simulink model "GridN3"  (R2021a)
settings: Solver=VariableStepAuto  StartTime=0.0  StopTime=10.0  RelTol=1e-3
libraries: spsDistributedParametersLineLib x22, spsThreePhaseSeriesRLCLoadLib x6, spsThreePhaseVIMeasurementLib x2, spspowerguiLib x1
settings Model: Creator=miair  LastModifiedBy=Admin
settings SolverCC: AlgebraicLoopSolver=TrustRegion
settings DataIOCC: ReturnWorkspaceOutputs=off
settings DebuggingCC: SFMachineParentedDataDiag=warning  ArithmeticOperatorsInVariantConditions=warning
settings SFSimCC: SimUseLocalCustomCode=off  CustomCodeUndefinedFunction=UseInterfaceOnly
settings RTWCC: RTWUseLocalCustomCode=off
settings CodeAppCC: StateflowObjectComments=on
settings SimscapeCC: SimscapeNormalizeSystem=off

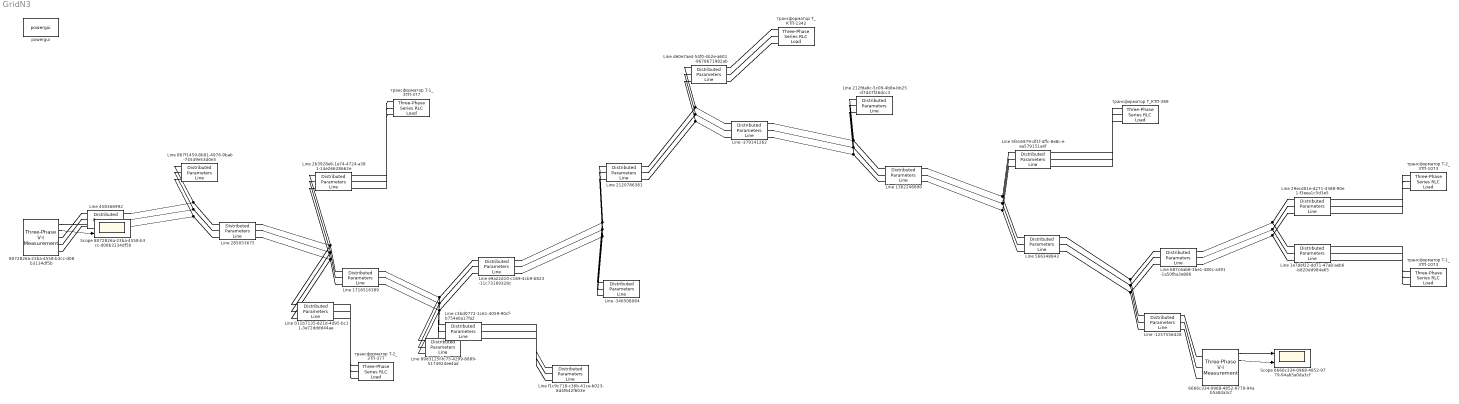
== system GridN3 ==
  6666c334-0968-4852-9779-94ab5a0da3cf : spsThreePhaseVIMeasurementLib/Three-Phase V-I Measurement  VoltageMeasurement=phase-to-ground  SetLabelV=off  LabelV=Vabc  Vpu=off  VpuLL=off  CurrentMeasurement=yes  SetLabelI=off  LabelI=Iabc  Ipu=off  Pbase=100e6  Vbase=500e3  OutputType=Complex  PhasorSimulation=on  PSBequivalent=0
  8072826a-23ba-4558-b3cc-d08b3134df5b : spsThreePhaseVIMeasurementLib/Three-Phase V-I Measurement  VoltageMeasurement=phase-to-ground  SetLabelV=off  LabelV=Vabc  Vpu=off  VpuLL=off  CurrentMeasurement=yes  SetLabelI=off  LabelI=Iabc  Ipu=off  Pbase=100e6  Vbase=500e3  OutputType=Complex  PhasorSimulation=on  PSBequivalent=0
  Line -1257556428 : spsDistributedParametersLineLib/Distributed Parameters Line  Description=Line connected to devices: [Опора-7/3_РВА-18-10кВ, ВВ РВА-19-10кВ]  Phases=3  Length=0.083645  Frequency=50  Resistance=[0.646656091154803 0.0486237908083191 0.0486712220507153;0.0486237908083191 0.646561225344642 0.0486237934466192;0.0486712220507153 0.0486237934466192 0.646656091154803]  Inductance=[0.00282448912315926 0.00133270803418135 0.00132951476746136;0.00133270803418135 0.00282479813276775 0.00133799988507366;0.00132951476746136 0.00133799988507366 0.00282448912315926]  Capacitance=[7.89543174552926e-09 -1.85986777702161e-09 -1.7901190036642e-09;-1.85986777702161e-09 7.82540023894543e-09 -1.8957321828871e-09;-1.7901190036642e-09 -1.8957321828871e-09 7.91264394645417e-09]  x1=[85.8130478893877 6561.48353456322 6560.92029844219;314.159265358979 314.159265358979 314.159265358979;0.298986720881434 -0.899555226132864 -2.47049778639167]  x2=[85.8130485695924 6561.4835673883 6560.92033132697;314.159265358979 314.159265358979 314.159265358979;0.298986717463087 -0.899555232497847 -2.47049779281051]  x3=[0.07502629314561 16.6966616361443 16.8234452112218;314.159265358979 314.159265358979 314.159265358979;0.298860809828188 -0.899655256227905 -2.47059791172944]  x4=[0.0750262931601746 16.6966616361894 16.8234452113946;314.159265358979 314.159265358979 314.159265358979;0.298986717302174 -0.899555232500781 -2.47049779281513]  x5=4.00782735046359e-07  V1=ones(3,3)  V2=ones(3,3)  I1=ones(3,3)  I2=ones(3,3)  nHarmo=1  Measurements=None  Decoupling=off  VsMag0=0  VrMag0=0  VsAngle0=0  VrAngle0=0  IsMag0=0  IrMag0=0  IsAngle0=0  IrAngle0=0
      settings: SourceProductBaseCode=PS
  Line -346508084 : spsDistributedParametersLineLib/Distributed Parameters Line  Description=Line connected to devices: [Опора-2/18_РВА-18-10кВ, трансформатор Т_ТП-1060]  Phases=3  Length=0.088705  Frequency=50  Resistance=[0.991907494602668 0.595664141602668 0.595664141602668;0.595664141602668 0.991907494602668 0.595664141602668;0.595664141602668 0.595664141602668 0.991907494602668]  Inductance=[0.0013307605340619 0.0010400448682494 0.0010400448682494;0.0010400448682494 0.0013307605340619 0.0010400448682494;0.0010400448682494 0.0010400448682494 0.0013307605340619]  Capacitance=[4.05772665830295e-07 -7.83285059789075e-08 -7.83285016498931e-08;-7.83285059789075e-08 4.05772632089447e-07 -7.83285164513028e-08;-7.83285016498931e-08 -7.83285164513028e-08 4.05772808751434e-07]  x1=[0.325825360935298 6568.42511930154 6568.48441213397;314.159265358979 314.159265358979 314.159265358979;0.746760518849295 2.95396210897823 1.38316414063238]  x2=[0.325825468435743 6568.42547824959 6568.48477108536;314.159265358979 314.159265358979 314.159265358979;0.746759846634459 2.95396187188771 1.3831639035418]  x3=[0.00278109088771278 267.749063807252 267.751511330739;314.159265358979 314.159265358979 314.159265358979;0.745947870811163 2.95363139241199 1.38283342402768]  x4=[0.00278109087609533 267.749063812641 267.751511335979;314.159265358979 314.159265358979 314.159265358979;0.746759838440762 2.95396187188745 1.38316390354211]  x5=2.58571089417873e-06  V1=ones(3,3)  V2=ones(3,3)  I1=ones(3,3)  I2=ones(3,3)  nHarmo=1  Measurements=None  Decoupling=off  VsMag0=0  VrMag0=0  VsAngle0=0  VrAngle0=0  IsMag0=0  IrMag0=0  IsAngle0=0  IrAngle0=0
      settings: SourceProductBaseCode=PS
  Line -379141262 : spsDistributedParametersLineLib/Distributed Parameters Line  Description=Line connected to devices: [Опора-2/22_РВА-18-10кВ, СШ ЗТП-921]  Phases=3  Length=0.22086  Frequency=50  Resistance=[0.646656091154803 0.0486237908083191 0.0486712220507153;0.0486237908083191 0.646561225344642 0.0486237934466192;0.0486712220507153 0.0486237934466192 0.646656091154803]  Inductance=[0.00282448912315926 0.00133270803418135 0.00132951476746136;0.00133270803418135 0.00282479813276775 0.00133799988507366;0.00132951476746136 0.00133799988507366 0.00282448912315926]  Capacitance=[7.89543174552926e-09 -1.85986777702161e-09 -1.7901190036642e-09;-1.85986777702161e-09 7.82540023894543e-09 -1.8957321828871e-09;-1.7901190036642e-09 -1.8957321828871e-09 7.91264394645417e-09]  x1=[85.7807223973082 6566.46218095662 6565.89154860446;314.159265358979 314.159265358979 314.159265358979;0.2985403295409 -0.899438697475493 -2.47038427952299]  x2=[85.7923784155305 6564.66837221298 6564.10040565809;314.159265358979 314.159265358979 314.159265358979;0.29862678418753 -0.899539931779373 -2.47048448218466]  x3=[0.104287106341695 6.82361878036728 6.92958778579486;314.159265358979 314.159265358979 314.159265358979;0.117621774807592 -0.363172627151027 -1.9436572281585]  x4=[0.0509827963357022 27.7636713522879 27.8913212019681;314.159265358979 314.159265358979 314.159265358979;0.675072542911708 -1.02556648080429 -2.59583033227613]  x5=1.0582446633073e-06  V1=ones(3,3)  V2=ones(3,3)  I1=ones(3,3)  I2=ones(3,3)  nHarmo=1  Measurements=None  Decoupling=off  VsMag0=0  VrMag0=0  VsAngle0=0  VrAngle0=0  IsMag0=0  IrMag0=0  IsAngle0=0  IrAngle0=0
      settings: SourceProductBaseCode=PS
  Line 011b7135-821d-4d95-bc11-3e72dddd44ae : spsDistributedParametersLineLib/Distributed Parameters Line  Description=Line connected to devices: [СШ ЗТП-377, трансформатор Т-2_ЗТП-377]  Phases=3  Length=0.005  Frequency=50  Resistance=[0.476003738225748 0.351747138225748 0.351747138225748;0.351747138225748 0.476003738225748 0.351747138225748;0.351747138225748 0.351747138225748 0.476003738225748]  Inductance=[0.000705954362986426 0.000459934243504405 0.000459934243504405;0.000459934243504405 0.000705954362986426 0.000459934243504405;0.000459934243504405 0.000459934243504405 0.000705954362986426]  Capacitance=[5.7561313269996e-07 -1.37543883484145e-07 -1.37543912800485e-07;-1.37543883484145e-07 5.75613027339387e-07 -1.37543875208088e-07;-1.37543912800485e-07 -1.37543875208088e-07 5.75613005057695e-07]  x1=[0.18202648425754 6574.92237471971 6574.93859363999;314.159265358979 314.159265358979 314.159265358979;0.731824412238409 -0.817080733458179 -2.38787252861853]  x2=[0.182026484492195 6574.92000203471 6574.93622094912;314.159265358979 314.159265358979 314.159265358979;0.731824413700631 -0.817080821744966 -2.38787261690532]  x3=[0.00247469117336317 350.815663562059 350.816501570652;314.159265358979 314.159265358979 314.159265358979;0.731816309663396 -0.81412926345355 -2.38492105836423]  x4=[0.0024745921934232 357.160743494514 357.161597181016;314.159265358979 314.159265358979 314.159265358979;0.731797613463593 -0.820000478759535 -2.39079227415924]  x5=1.10521588109605e-07  V1=ones(3,3)  V2=ones(3,3)  I1=ones(3,3)  I2=ones(3,3)  nHarmo=1  Measurements=None  Decoupling=off  VsMag0=0  VrMag0=0  VsAngle0=0  VrAngle0=0  IsMag0=0  IrMag0=0  IsAngle0=0  IrAngle0=0
      settings: SourceProductBaseCode=PS
  Line 1362246896 : spsDistributedParametersLineLib/Distributed Parameters Line  Description=Line connected to devices: [СШ ЗТП-921, СШ КТП-389]  Phases=3  Length=0.37012  Frequency=50  Resistance=[0.646656091154803 0.0486237908083191 0.0486712220507153;0.0486237908083191 0.646561225344642 0.0486237934466192;0.0486712220507153 0.0486237934466192 0.646656091154803]  Inductance=[0.00282448912315926 0.00133270803418135 0.00132951476746136;0.00133270803418135 0.00282479813276775 0.00133799988507366;0.00132951476746136 0.00133799988507366 0.00282448912315926]  Capacitance=[7.89543174552926e-09 -1.85986777702161e-09 -1.7901190036642e-09;-1.85986777702161e-09 7.82540023894543e-09 -1.8957321828871e-09;-1.7901190036642e-09 -1.8957321828871e-09 7.91264394645417e-09]  x1=[85.7923784155308 6564.66837221298 6564.10040565809;314.159265358979 314.159265358979 314.159265358979;0.298402105266729 -0.899718424425486 -2.47066314474314]  x2=[85.8119032777789 6561.66012948809 6561.09663330914;314.159265358979 314.159265358979 314.159265358979;0.298546930444211 -0.899887751165177 -2.47083073957211]  x3=[0.104282336760185 6.82326507299442 6.92908966322945;314.159265358979 314.159265358979 314.159265358979;0.11750414593762 -0.361669324534678 -1.94217067702694]  x4=[0.0509963380008713 27.7541994828913 27.8817464459583;314.159265358979 314.159265358979 314.159265358979;0.674503619209762 -1.02641198177557 -2.59667506905694]  x5=1.77341988039164e-06  V1=ones(3,3)  V2=ones(3,3)  I1=ones(3,3)  I2=ones(3,3)  nHarmo=1  Measurements=None  Decoupling=off  VsMag0=0  VrMag0=0  VsAngle0=0  VrAngle0=0  IsMag0=0  IrMag0=0  IsAngle0=0  IrAngle0=0
      settings: SourceProductBaseCode=PS
  Line 1716516389 : spsDistributedParametersLineLib/Distributed Parameters Line  Description=Line connected to devices: [СШ ЗТП-377, Опора-2/17_РВА-18-10кВ]  Phases=3  Length=0.75608  Frequency=50  Resistance=[0.646656091154803 0.0486237908083191 0.0486712220507153;0.0486237908083191 0.646561225344642 0.0486237934466192;0.0486712220507153 0.0486237934466192 0.646656091154803]  Inductance=[0.00282448912315926 0.00133270803418135 0.00132951476746136;0.00133270803418135 0.00282479813276775 0.00133799988507366;0.00132951476746136 0.00133799988507366 0.00282448912315926]  Capacitance=[7.89543174552926e-09 -1.85986777702161e-09 -1.7901190036642e-09;-1.85986777702161e-09 7.82540023894543e-09 -1.8957321828871e-09;-1.7901190036642e-09 -1.8957321828871e-09 7.91264394645417e-09]  x1=[85.7303472897462 6574.23848711095 6573.65682525224;314.159265358979 314.159265358979 314.159265358979;0.297343931698933 -0.899609585013276 -2.47056030786269]  x2=[85.7698176529276 6568.14269532905 6567.56961227306;314.159265358979 314.159265358979 314.159265358979;0.297652273334468 -0.899981244223213 -2.47092840739886]  x3=[0.10467535670815 6.59358891496528 6.70130181002506;314.159265358979 314.159265358979 314.159265358979;0.122437480289168 -0.392072680443273 -1.97247119055127]  x4=[0.0502114079757094 27.8421642336423 27.9697944201387;314.159265358979 314.159265358979 314.159265358979;0.667253673963557 -1.01573694491228 -2.58604709943669]  x5=3.62273668855104e-06  V1=ones(3,3)  V2=ones(3,3)  I1=ones(3,3)  I2=ones(3,3)  nHarmo=1  Measurements=None  Decoupling=off  VsMag0=0  VrMag0=0  VsAngle0=0  VrAngle0=0  IsMag0=0  IrMag0=0  IsAngle0=0  IrAngle0=0
      settings: SourceProductBaseCode=PS
  Line 1e7def22-dd71-47a8-aeb6-b820dd984e65 : spsDistributedParametersLineLib/Distributed Parameters Line  Description=Line connected to devices: [СШ ЗТП-1073, трансформатор Т-1_ЗТП-1073]  Phases=3  Length=0.005  Frequency=50  Resistance=[0.476003738225748 0.351747138225748 0.351747138225748;0.351747138225748 0.476003738225748 0.351747138225748;0.351747138225748 0.351747138225748 0.476003738225748]  Inductance=[0.000705954362986426 0.000459934243504405 0.000459934243504405;0.000459934243504405 0.000705954362986426 0.000459934243504405;0.000459934243504405 0.000459934243504405 0.000705954362986426]  Capacitance=[5.7561313269996e-07 -1.37543883484145e-07 -1.37543912800485e-07;-1.37543883484145e-07 5.75613027339387e-07 -1.37543875208088e-07;-1.37543912800485e-07 -1.37543875208088e-07 5.75613005057695e-07]  x1=[0.457408916025327 6562.02369079989 6562.06425701034;314.159265358979 314.159265358979 314.159265358979;0.736293928023844 -0.817827314983347 -2.38861215687802]  x2=[0.457408916407412 6562.02166126246 6562.06222746036;314.159265358979 314.159265358979 314.159265358979;0.736293927567955 -0.817827390707452 -2.38861223260212]  x3=[0.0062184945191106 350.579364851524 350.581504811006;314.159265358979 314.159265358979 314.159265358979;0.736267900596507 -0.815303741071734 -2.38608858275119]  x4=[0.00621841215540893 356.007341807378 356.009515319894;314.159265358979 314.159265358979 314.159265358979;0.736285117710504 -0.820333135503826 -2.39111797759822]  x5=1.10521588109605e-07  V1=ones(3,3)  V2=ones(3,3)  I1=ones(3,3)  I2=ones(3,3)  nHarmo=1  Measurements=None  Decoupling=off  VsMag0=0  VrMag0=0  VsAngle0=0  VrAngle0=0  IsMag0=0  IrMag0=0  IsAngle0=0  IrAngle0=0
      settings: SourceProductBaseCode=PS
  Line 2120786381 : spsDistributedParametersLineLib/Distributed Parameters Line  Description=Line connected to devices: [Опора-2/18_РВА-18-10кВ, Опора-2/22_РВА-18-10кВ]  Phases=3  Length=0.1588  Frequency=50  Resistance=[0.646656091154803 0.0486237908083191 0.0486712220507153;0.0486237908083191 0.646561225344642 0.0486237934466192;0.0486712220507153 0.0486237934466192 0.646656091154803]  Inductance=[0.00282448912315926 0.00133270803418135 0.00132951476746136;0.00133270803418135 0.00282479813276775 0.00133799988507366;0.00132951476746136 0.00133799988507366 0.00282448912315926]  Capacitance=[7.89543174552926e-09 -1.85986777702161e-09 -1.7901190036642e-09;-1.85986777702161e-09 7.82540023894543e-09 -1.8957321828871e-09;-1.7901190036642e-09 -1.8957321828871e-09 7.91264394645417e-09]  x1=[85.7723025572561 6567.75932160512 6567.18679065402;314.159265358979 314.159265358979 314.159265358979;0.298570352621644 -0.899289613819206 -2.4702358745204]  x2=[85.7807223973084 6566.46218095662 6565.89154860446;314.159265358979 314.159265358979 314.159265358979;0.298633747561971 -0.899364482993263 -2.47030999439383]  x3=[0.104648648733326 6.69890268386915 6.80472766998649;314.159265358979 314.159265358979 314.159265358979;0.118499232296056 -0.360864666108681 -1.94157017108293]  x4=[0.0506190945789256 27.8809412809424 28.0086787475238;314.159265358979 314.159265358979 314.159265358979;0.677585502188691 -1.02296914278802 -2.59324453503301]  x5=7.6088586676265e-07  V1=ones(3,3)  V2=ones(3,3)  I1=ones(3,3)  I2=ones(3,3)  nHarmo=1  Measurements=None  Decoupling=off  VsMag0=0  VrMag0=0  VsAngle0=0  VrAngle0=0  IsMag0=0  IrMag0=0  IsAngle0=0  IrAngle0=0
      settings: SourceProductBaseCode=PS
  Line 212fda6c-5c09-4b8e-bb25-d7d47f26dcc3 : spsDistributedParametersLineLib/Distributed Parameters Line  Description=Line connected to devices: [СШ ЗТП-921, разъединитель ЗТП-921]  Phases=3  Length=0.005  Frequency=50  Resistance=[0.476003738225748 0.351747138225748 0.351747138225748;0.351747138225748 0.476003738225748 0.351747138225748;0.351747138225748 0.351747138225748 0.476003738225748]  Inductance=[0.000705954362986426 0.000459934243504405 0.000459934243504405;0.000459934243504405 0.000705954362986426 0.000459934243504405;0.000459934243504405 0.000459934243504405 0.000705954362986426]  Capacitance=[5.7561313269996e-07 -1.37543883484145e-07 -1.37543912800485e-07;-1.37543883484145e-07 5.75613027339387e-07 -1.37543875208088e-07;-1.37543912800485e-07 -1.37543875208088e-07 5.75613005057695e-07]  x1=[0.389068788758442 6565.34837754689 6565.38275121948;314.159265358979 314.159265358979 314.159265358979;0.738193501479332 -0.817650989189443 -2.38843755120427]  x2=[0.389068788992651 6565.34837896798 6565.38275264058;314.159265358979 314.159265358979 314.159265358979;0.738193500098076 -0.817650989537432 -2.38843755155226]  x3=[0.00528937246271574 353.471288570416 353.47311190086;314.159265358979 314.159265358979 314.159265358979;0.738158905285153 -0.817671795792498 -2.38845835780669]  x4=[0.00528937260697671 353.47128859302 353.47311189454;314.159265358979 314.159265358979 314.159265358979;0.738193290271334 -0.817650989550849 -2.38843755155911]  x5=1.10521588109605e-07  V1=ones(3,3)  V2=ones(3,3)  I1=ones(3,3)  I2=ones(3,3)  nHarmo=1  Measurements=None  Decoupling=off  VsMag0=0  VrMag0=0  VsAngle0=0  VrAngle0=0  IsMag0=0  IrMag0=0  IsAngle0=0  IrAngle0=0
      settings: SourceProductBaseCode=PS
  Line 285053675 : spsDistributedParametersLineLib/Distributed Parameters Line  Description=Line connected to devices: [Опора-1/6_РВА-18-10кВ, СШ ЗТП-377]  Phases=3  Length=0.3882  Frequency=50  Resistance=[0.646656091154803 0.0486237908083191 0.0486712220507153;0.0486237908083191 0.646561225344642 0.0486237934466192;0.0486712220507153 0.0486237934466192 0.646656091154803]  Inductance=[0.00282448912315926 0.00133270803418135 0.00132951476746136;0.00133270803418135 0.00282479813276775 0.00133799988507366;0.00132951476746136 0.00133799988507366 0.00282448912315926]  Capacitance=[7.89543174552926e-09 -1.85986777702161e-09 -1.7901190036642e-09;-1.85986777702161e-09 7.82540023894543e-09 -1.8957321828871e-09;-1.7901190036642e-09 -1.8957321828871e-09 7.91264394645417e-09]  x1=[85.6980498781803 6579.21748277583 6578.62863320459;314.159265358979 314.159265358979 314.159265358979;0.297650542376148 -0.89887590056258 -2.46982908698223]  x2=[85.7303472897462 6574.23848711095 6573.65682525224;314.159265358979 314.159265358979 314.159265358979;0.297897696146105 -0.899169655530145 -2.47011995959784]  x3=[0.122743715524074 5.30429248137885 5.28780830142103;314.159265358979 314.159265358979 314.159265358979;0.0571706483292508 0.778310934748027 -0.815772719494164]  x4=[0.0423356221015817 34.4308758330315 34.5589745167785;314.159265358979 314.159265358979 314.159265358979;1.05903750527836 -1.05303932289333 -2.62327728965936]  x5=1.86004970703565e-06  V1=ones(3,3)  V2=ones(3,3)  I1=ones(3,3)  I2=ones(3,3)  nHarmo=1  Measurements=None  Decoupling=off  VsMag0=0  VrMag0=0  VsAngle0=0  VrAngle0=0  IsMag0=0  IrMag0=0  IsAngle0=0  IrAngle0=0
      settings: SourceProductBaseCode=PS
  Line 29ecd01e-d271-4388-90e1-f3eea1c5d3e5 : spsDistributedParametersLineLib/Distributed Parameters Line  Description=Line connected to devices: [СШ ЗТП-1073, трансформатор Т-2_ЗТП-1073]  Phases=3  Length=0.005  Frequency=50  Resistance=[0.476003738225748 0.351747138225748 0.351747138225748;0.351747138225748 0.476003738225748 0.351747138225748;0.351747138225748 0.351747138225748 0.476003738225748]  Inductance=[0.000705954362986426 0.000459934243504405 0.000459934243504405;0.000459934243504405 0.000705954362986426 0.000459934243504405;0.000459934243504405 0.000459934243504405 0.000705954362986426]  Capacitance=[5.7561313269996e-07 -1.37543883484145e-07 -1.37543912800485e-07;-1.37543883484145e-07 5.75613027339387e-07 -1.37543875208088e-07;-1.37543912800485e-07 -1.37543875208088e-07 5.75613005057695e-07]  x1=[0.457408916025327 6562.02369079989 6562.06425701034;314.159265358979 314.159265358979 314.159265358979;0.736293928023844 -0.817827314983347 -2.38861215687802]  x2=[0.457408916410203 6562.02166126246 6562.06222746036;314.159265358979 314.159265358979 314.159265358979;0.736293927590602 -0.817827390707452 -2.38861223260212]  x3=[0.00621849586382799 350.579364858309 350.581504810186;314.159265358979 314.159265358979 314.159265358979;0.736268171375189 -0.815303741069756 -2.3860885827578]  x4=[0.00621841124335336 356.007341800217 356.009515320748;314.159265358979 314.159265358979 314.159265358979;0.736284988079895 -0.820333135504027 -2.39111797759029]  x5=1.10521588109605e-07  V1=ones(3,3)  V2=ones(3,3)  I1=ones(3,3)  I2=ones(3,3)  nHarmo=1  Measurements=None  Decoupling=off  VsMag0=0  VrMag0=0  VsAngle0=0  VrAngle0=0  IsMag0=0  IrMag0=0  IsAngle0=0  IrAngle0=0
      settings: SourceProductBaseCode=PS
  Line 2b3928e6-1e74-4724-a381-14e26628662e : spsDistributedParametersLineLib/Distributed Parameters Line  Description=Line connected to devices: [СШ ЗТП-377, трансформатор Т-1_ЗТП-377]  Phases=3  Length=0.005  Frequency=50  Resistance=[0.476003738225748 0.351747138225748 0.351747138225748;0.351747138225748 0.476003738225748 0.351747138225748;0.351747138225748 0.351747138225748 0.476003738225748]  Inductance=[0.000705954362986426 0.000459934243504405 0.000459934243504405;0.000459934243504405 0.000705954362986426 0.000459934243504405;0.000459934243504405 0.000459934243504405 0.000705954362986426]  Capacitance=[5.7561313269996e-07 -1.37543883484145e-07 -1.37543912800485e-07;-1.37543883484145e-07 5.75613027339387e-07 -1.37543875208088e-07;-1.37543912800485e-07 -1.37543875208088e-07 5.75613005057695e-07]  x1=[0.18202648425754 6574.92237471971 6574.93859363999;314.159265358979 314.159265358979 314.159265358979;0.731824412238409 -0.817080733458179 -2.38787252861853]  x2=[0.182026484492417 6574.92000203471 6574.93622094912;314.159265358979 314.159265358979 314.159265358979;0.731824413686101 -0.817080821744966 -2.38787261690532]  x3=[0.00247469079372481 350.81566355941 350.816501566115;314.159265358979 314.159265358979 314.159265358979;0.731816301440955 -0.814129263441908 -2.38492105837358]  x4=[0.00247459218329001 357.160743496938 357.161597185482;314.159265358979 314.159265358979 314.159265358979;0.731797690177833 -0.820000478772449 -2.39079227414992]  x5=1.10521588109605e-07  V1=ones(3,3)  V2=ones(3,3)  I1=ones(3,3)  I2=ones(3,3)  nHarmo=1  Measurements=None  Decoupling=off  VsMag0=0  VrMag0=0  VsAngle0=0  VrAngle0=0  IsMag0=0  IrMag0=0  IsAngle0=0  IrAngle0=0
      settings: SourceProductBaseCode=PS
  Line 458366992 : spsDistributedParametersLineLib/Distributed Parameters Line  Description=Line connected to devices: [ВВ РВА-18-10кВ, Опора-1/6_РВА-18-10кВ]  Phases=3  Length=0.26932  Frequency=50  Resistance=[0.646656091154803 0.0486237908083191 0.0486712220507153;0.0486237908083191 0.646561225344642 0.0486237934466192;0.0486712220507153 0.0486237934466192 0.646656091154803]  Inductance=[0.00282448912315926 0.00133270803418135 0.00132951476746136;0.00133270803418135 0.00282479813276775 0.00133799988507366;0.00132951476746136 0.00133799988507366 0.00282448912315926]  Capacitance=[7.89543174552926e-09 -1.85986777702161e-09 -1.7901190036642e-09;-1.85986777702161e-09 7.82540023894543e-09 -1.8957321828871e-09;-1.7901190036642e-09 -1.8957321828871e-09 7.91264394645417e-09]  x1=[85.6756288761045 6582.67123992655 6582.0773957145;314.159265358979 314.159265358979 314.159265358979;0.297658001031491 -0.898530040368513 -2.4694850868605]  x2=[85.6980498781802 6579.21748277583 6578.62863320459;314.159265358979 314.159265358979 314.159265358979;0.297829490722023 -0.898733737854755 -2.46968678894557]  x3=[0.122741132978438 5.30178361506566 5.28545786297625;314.159265358979 314.159265358979 314.159265358979;0.0569718092663794 0.776703130031307 -0.817410056242542]  x4=[0.0423353625676533 34.4453096076244 34.5735345578591;314.159265358979 314.159265358979 314.159265358979;1.06008637954097 -1.05247314760449 -2.6227108080572]  x5=1.29043943096043e-06  V1=ones(3,3)  V2=ones(3,3)  I1=ones(3,3)  I2=ones(3,3)  nHarmo=1  Measurements=None  Decoupling=off  VsMag0=0  VrMag0=0  VsAngle0=0  VrAngle0=0  IsMag0=0  IrMag0=0  IsAngle0=0  IrAngle0=0
      settings: SourceProductBaseCode=PS
  Line 566348843 : spsDistributedParametersLineLib/Distributed Parameters Line  Description=Line connected to devices: [СШ КТП-389, Опора-7/3_РВА-18-10кВ]  Phases=3  Length=0.043512  Frequency=50  Resistance=[0.646656091154803 0.0486237908083191 0.0486712220507153;0.0486237908083191 0.646561225344642 0.0486237934466192;0.0486712220507153 0.0486237934466192 0.646656091154803]  Inductance=[0.00282448912315926 0.00133270803418135 0.00132951476746136;0.00133270803418135 0.00282479813276775 0.00133799988507366;0.00132951476746136 0.00133799988507366 0.00282448912315926]  Capacitance=[7.89543174552926e-09 -1.85986777702161e-09 -1.7901190036642e-09;-1.85986777702161e-09 7.82540023894543e-09 -1.8957321828871e-09;-1.7901190036642e-09 -1.8957321828871e-09 7.91264394645417e-09]  x1=[85.8119032777789 6561.66012948809 6561.09663330914;314.159265358979 314.159265358979 314.159265358979;0.299038568746273 -0.899497176824017 -2.47043979343183]  x2=[85.8130478893877 6561.48353456322 6560.92029844219;314.159265358979 314.159265358979 314.159265358979;0.299047132506305 -0.899507233064618 -2.47044974763742]  x3=[0.0893414801134547 11.4015000518715 11.5255435179219;314.159265358979 314.159265358979 314.159265358979;0.194545547128172 -0.747199547146555 -2.31991390560546]  x4=[0.061905075390855 22.193362297922 22.3207748538051;314.159265358979 314.159265358979 314.159265358979;0.450073304452099 -0.97756162265115 -2.54799656571274]  x5=2.08486560671136e-07  V1=ones(3,3)  V2=ones(3,3)  I1=ones(3,3)  I2=ones(3,3)  nHarmo=1  Measurements=None  Decoupling=off  VsMag0=0  VrMag0=0  VsAngle0=0  VrAngle0=0  IsMag0=0  IrMag0=0  IsAngle0=0  IrAngle0=0
      settings: SourceProductBaseCode=PS
  Line 5fe16979-df1f-4ffc-8e8c-eea579151a4f : spsDistributedParametersLineLib/Distributed Parameters Line  Description=Line connected to devices: [СШ КТП-389, трансформатор Т_КТП-389]  Phases=3  Length=0.005  Frequency=50  Resistance=[0.476003738225748 0.351747138225748 0.351747138225748;0.351747138225748 0.476003738225748 0.351747138225748;0.351747138225748 0.351747138225748 0.476003738225748]  Inductance=[0.000705954362986426 0.000459934243504405 0.000459934243504405;0.000459934243504405 0.000705954362986426 0.000459934243504405;0.000459934243504405 0.000459934243504405 0.000705954362986426]  Capacitance=[5.7561313269996e-07 -1.37543883484145e-07 -1.37543912800485e-07;-1.37543883484145e-07 5.75613027339387e-07 -1.37543875208088e-07;-1.37543912800485e-07 -1.37543875208088e-07 5.75613005057695e-07]  x1=[0.45361470502657 6562.33892407618 6562.37914965594;314.159265358979 314.159265358979 314.159265358979;0.736354846822467 -0.817820271602062 -2.38860520926576]  x2=[0.453614705521787 6562.33487354237 6562.3750990973;314.159265358979 314.159265358979 314.159265358979;0.736354847365546 -0.817820422325358 -2.38860535998905]  x3=[0.00616695780949283 347.8990046977 347.901109930978;314.159265358979 314.159265358979 314.159265358979;0.73633809286147 -0.812725669015981 -2.3835106062512]  x4=[0.00616678641523404 358.728232821492 358.730404420506;314.159265358979 314.159265358979 314.159265358979;0.736336689311416 -0.822781718907569 -2.39356665696539]  x5=1.10521588109605e-07  V1=ones(3,3)  V2=ones(3,3)  I1=ones(3,3)  I2=ones(3,3)  nHarmo=1  Measurements=None  Decoupling=off  VsMag0=0  VrMag0=0  VsAngle0=0  VrAngle0=0  IsMag0=0  IrMag0=0  IsAngle0=0  IrAngle0=0
      settings: SourceProductBaseCode=PS
  Line 687c6ab8-3be1-480c-a391-1a50fba3e886 : spsDistributedParametersLineLib/Distributed Parameters Line  Description=Line connected to devices: [Опора-7/3_РВА-18-10кВ, СШ ЗТП-1073]  Phases=3  Length=0.043769  Frequency=50  Resistance=[1.20319872737733 0.650615891377333 0.650615891377333;0.650615891377333 1.20319872737733 0.650615891377333;0.650615891377333 0.650615891377333 1.20319872737733]  Inductance=[0.00152224047491712 0.00121971605345402 0.00121971605345402;0.00121971605345402 0.00152224047491712 0.00121971605345402;0.00121971605345402 0.00121971605345402 0.00152224047491712]  Capacitance=[3.5492678521701e-07 -6.81668751215391e-08 -6.81669173453455e-08;-6.81668751215391e-08 3.54926826597295e-07 -6.81668989311185e-08;-6.81669173453455e-08 -6.81668989311185e-08 3.5492692272688e-07]  x1=[0.458696725832891 6562.14016601679 6562.22491666675;314.159265358979 314.159265358979 314.159265358979;0.743269903598006 -0.209383378081335 1.361411125857]  x2=[0.458696776784068 6562.00159936247 6562.08634822285;314.159265358979 314.159265358979 314.159265358979;0.743269546706823 -0.209380367796599 1.36141413614169]  x3=[0.00340495238839209 239.819205901043 239.822338500464;314.159265358979 314.159265358979 314.159265358979;0.742661547688956 -0.202167578861455 1.36862692394507]  x4=[0.00340539683050802 250.665435075402 250.668707755741;314.159265358979 314.159265358979 314.159265358979;0.7434731225717 -0.216436236026366 1.35435826892828]  x5=1.28802439821471e-06  V1=ones(3,3)  V2=ones(3,3)  I1=ones(3,3)  I2=ones(3,3)  nHarmo=1  Measurements=None  Decoupling=off  VsMag0=0  VrMag0=0  VsAngle0=0  VrAngle0=0  IsMag0=0  IrMag0=0  IsAngle0=0  IrAngle0=0
      settings: SourceProductBaseCode=PS
  Line 867f1459-8b81-4976-9bab-74549e53d0e3 : spsDistributedParametersLineLib/Distributed Parameters Line  Description=Line connected to devices: [Опора-1/6_РВА-18-10кВ, трансформатор КТП-881]  Phases=3  Length=0.00065343  Frequency=50  Resistance=[0.646656091154803 0.0486237908083191 0.0486712220507153;0.0486237908083191 0.646561225344642 0.0486237934466192;0.0486712220507153 0.0486237934466192 0.646656091154803]  Inductance=[0.00282448912315926 0.00133270803418135 0.00132951476746136;0.00133270803418135 0.00282479813276775 0.00133799988507366;0.00132951476746136 0.00133799988507366 0.00282448912315926]  Capacitance=[7.89543174552926e-09 -1.85986777702161e-09 -1.7901190036642e-09;-1.85986777702161e-09 7.82540023894543e-09 -1.8957321828871e-09;-1.7901190036642e-09 -1.8957321828871e-09 7.91264394645417e-09]  x1=[85.6980498781803 6579.21748277583 6578.62863320459;314.159265358979 314.159265358979 314.159265358979;0.298233910626906 -0.898412452801818 -2.46936519805201]  x2=[85.6980498782296 6579.21748277784 6578.6286332066;314.159265358979 314.159265358979 314.159265358979;0.298233910626714 -0.898412452802205 -2.4693651980524]  x3=[0.0749287810848881 16.7433737787774 16.8704622471718;314.159265358979 314.159265358979 314.159265358979;0.298232846373062 -0.898413233666011 -2.46936597954687]  x4=[0.074928772237256 16.7433737557272 16.8704622525088;314.159265358979 314.159265358979 314.159265358979;0.298233984208292 -0.898412453300088 -2.46936519860446]  x5=3.1308920146015e-09  V1=ones(3,3)  V2=ones(3,3)  I1=ones(3,3)  I2=ones(3,3)  nHarmo=1  Measurements=None  Decoupling=off  VsMag0=0  VrMag0=0  VsAngle0=0  VrAngle0=0  IsMag0=0  IrMag0=0  IsAngle0=0  IrAngle0=0
      settings: SourceProductBaseCode=PS
  Line 89d3125f-fc75-4299-8889-5174924ee4ad : spsDistributedParametersLineLib/Distributed Parameters Line  Description=Line connected to devices: [Опора-2/17_РВА-18-10кВ, трансформатор Т_КТП-1374]  Phases=3  Length=0.0029735  Frequency=50  Resistance=[0.991907494602668 0.595664141602668 0.595664141602668;0.595664141602668 0.991907494602668 0.595664141602668;0.595664141602668 0.595664141602668 0.991907494602668]  Inductance=[0.0013307605340619 0.0010400448682494 0.0010400448682494;0.0010400448682494 0.0013307605340619 0.0010400448682494;0.0010400448682494 0.0010400448682494 0.0013307605340619]  Capacitance=[4.05772665830295e-07 -7.83285059789075e-08 -7.83285016498931e-08;-7.83285059789075e-08 4.05772632089447e-07 -7.83285164513028e-08;-7.83285016498931e-08 -7.83285164513028e-08 4.05772808751434e-07]  x1=[0.317544050960836 6568.8090476792 6568.8668115264;314.159265358979 314.159265358979 314.159265358979;0.747727267190857 2.95430412100218 1.38350619486673]  x2=[0.31754405107292 6568.80904808256 6568.86681192977;314.159265358979 314.159265358979 314.159265358979;0.747727266448953 2.95430412073577 1.38350619460032]  x3=[0.00271365733041406 268.043215065309 268.045602780873;314.159265358979 314.159265358979 314.159265358979;0.747700614216486 2.954293038826 1.38349511268853]  x4=[0.00271365824520058 268.043215066634 268.045602775701;314.159265358979 314.159265358979 314.159265358979;0.747726830849994 2.9543041207267 1.38350619459306]  x5=8.66761889841661e-08  V1=ones(3,3)  V2=ones(3,3)  I1=ones(3,3)  I2=ones(3,3)  nHarmo=1  Measurements=None  Decoupling=off  VsMag0=0  VrMag0=0  VsAngle0=0  VrAngle0=0  IsMag0=0  IrMag0=0  IsAngle0=0  IrAngle0=0
      settings: SourceProductBaseCode=PS
  Line c3bd0772-1c61-4059-90cf-b754e0a17fa2 : spsDistributedParametersLineLib/Distributed Parameters Line  Description=Line connected to devices: [Опора-2/17_РВА-18-10кВ, разъединитель ЛР-235-10кВ]  Phases=3  Length=7.7673e-05  Frequency=50  Resistance=[0.646656091154803 0.0486237908083191 0.0486712220507153;0.0486237908083191 0.646561225344642 0.0486237934466192;0.0486712220507153 0.0486237934466192 0.646656091154803]  Inductance=[0.00282448912315926 0.00133270803418135 0.00132951476746136;0.00133270803418135 0.00282479813276775 0.00133799988507366;0.00132951476746136 0.00133799988507366 0.00282448912315926]  Capacitance=[7.89543174552926e-09 -1.85986777702161e-09 -1.7901190036642e-09;-1.85986777702161e-09 7.82540023894543e-09 -1.8957321828871e-09;-1.7901190036642e-09 -1.8957321828871e-09 7.91264394645417e-09]  x1=[85.7698176529277 6568.14269532905 6567.56961227306;314.159265358979 314.159265358979 314.159265358979;0.29879027271109 -0.899077178460024 -2.47002348102908]  x2=[85.7698176120966 6568.14269991505 6567.56961683061;314.159265358979 314.159265358979 314.159265358979;0.298790273108476 -0.899077179348645 -2.47002348191753]  x3=[0.0750962780064888 16.7156545226998 16.84259947248;314.159265358979 314.159265358979 314.159265358979;0.303452590994299 -0.906595501520112 -2.47748597400001]  x4=[0.0748885031924901 16.7156916115006 16.8425650066497;314.159265358979 314.159265358979 314.159265358979;0.29411462257478 -0.891558965801733 -2.46256106711389]  x5=3.72168060006646e-10  V1=ones(3,3)  V2=ones(3,3)  I1=ones(3,3)  I2=ones(3,3)  nHarmo=1  Measurements=None  Decoupling=off  VsMag0=0  VrMag0=0  VsAngle0=0  VrAngle0=0  IsMag0=0  IrMag0=0  IsAngle0=0  IrAngle0=0
      settings: SourceProductBaseCode=PS
  Line d60e7ae4-54f0-4b2e-a601-9678671982ab : spsDistributedParametersLineLib/Distributed Parameters Line  Description=Line connected to devices: [Опора-2/22_РВА-18-10кВ, трансформатор Т_КТП-1342]  Phases=3  Length=0.088295  Frequency=50  Resistance=[0.991907494602668 0.595664141602668 0.595664141602668;0.595664141602668 0.991907494602668 0.595664141602668;0.595664141602668 0.595664141602668 0.991907494602668]  Inductance=[0.0013307605340619 0.0010400448682494 0.0010400448682494;0.0010400448682494 0.0013307605340619 0.0010400448682494;0.0010400448682494 0.0010400448682494 0.0013307605340619]  Capacitance=[4.05772665830295e-07 -7.83285059789075e-08 -7.83285016498931e-08;-7.83285059789075e-08 4.05772632089447e-07 -7.83285164513028e-08;-7.83285016498931e-08 -7.83285164513028e-08 4.05772808751434e-07]  x1=[0.353759191864802 6567.12612735337 6567.19057310941;314.159265358979 314.159265358979 314.159265358979;0.745631420112232 2.95388921236969 1.3830910960456]  x2=[0.353759305861177 6567.12201039793 6567.18645611366;314.159265358979 314.159265358979 314.159265358979;0.74563075149158 2.95388903962976 1.38309092330563]  x3=[0.00301952940415001 267.578684824401 267.581341238932;314.159265358979 314.159265358979 314.159265358979;0.744822366440518 2.95370574591213 1.38290762953532]  x4=[0.00301954687901249 267.816013027388 267.818671770266;314.159265358979 314.159265358979 314.159265358979;0.745630907583076 2.95374330201086 1.38294518570168]  x5=2.5737595783948e-06  V1=ones(3,3)  V2=ones(3,3)  I1=ones(3,3)  I2=ones(3,3)  nHarmo=1  Measurements=None  Decoupling=off  VsMag0=0  VrMag0=0  VsAngle0=0  VrAngle0=0  IsMag0=0  IrMag0=0  IsAngle0=0  IrAngle0=0
      settings: SourceProductBaseCode=PS
  Line e9a22d10-c169-4cb9-b823-11c73169328c : spsDistributedParametersLineLib/Distributed Parameters Line  Description=Line connected to devices: [Опора-2/17_РВА-18-10кВ, Опора-2/18_РВА-18-10кВ]  Phases=3  Length=0.047179  Frequency=50  Resistance=[0.646656091154803 0.0486237908083191 0.0486712220507153;0.0486237908083191 0.646561225344642 0.0486237934466192;0.0486712220507153 0.0486237934466192 0.646656091154803]  Inductance=[0.00282448912315926 0.00133270803418135 0.00132951476746136;0.00133270803418135 0.00282479813276775 0.00133799988507366;0.00132951476746136 0.00133799988507366 0.00282448912315926]  Capacitance=[7.89543174552926e-09 -1.85986777702161e-09 -1.7901190036642e-09;-1.85986777702161e-09 7.82540023894543e-09 -1.8957321828871e-09;-1.7901190036642e-09 -1.8957321828871e-09 7.91264394645417e-09]  x1=[85.7698176529278 6568.14269532905 6567.56961227306;314.159265358979 314.159265358979 314.159265358979;0.298719371764295 -0.899133504605619 -2.47007986079318]  x2=[85.7723025572563 6567.75932160512 6567.18679065402;314.159265358979 314.159265358979 314.159265358979;0.298738374099725 -0.899156131790185 -2.47010226542594]  x3=[0.104681062942395 6.65562497957956 6.76224600986117;314.159265358979 314.159265358979 314.159265358979;0.121047810104768 -0.372364288212508 -1.95295517251809]  x4=[0.0504611288077385 27.8759779681348 28.0038076333477;314.159265358979 314.159265358979 314.159265358979;0.674032973096849 -1.01950554880495 -2.5897946062842]  x5=2.26056891108281e-07  V1=ones(3,3)  V2=ones(3,3)  I1=ones(3,3)  I2=ones(3,3)  nHarmo=1  Measurements=None  Decoupling=off  VsMag0=0  VrMag0=0  VsAngle0=0  VrAngle0=0  IsMag0=0  IrMag0=0  IsAngle0=0  IrAngle0=0
      settings: SourceProductBaseCode=PS
  Line f1c9c718-c36b-41ce-b023-8d4f642f603e : spsDistributedParametersLineLib/Distributed Parameters Line  Description=Line connected to devices: [разъединитель ЛР-235-10кВ, трансформатор Т_КТП-1303]  Phases=3  Length=0.12578  Frequency=50  Resistance=[0.991907494602668 0.595664141602668 0.595664141602668;0.595664141602668 0.991907494602668 0.595664141602668;0.595664141602668 0.595664141602668 0.991907494602668]  Inductance=[0.0013307605340619 0.0010400448682494 0.0010400448682494;0.0010400448682494 0.0013307605340619 0.0010400448682494;0.0010400448682494 0.0010400448682494 0.0013307605340619]  Capacitance=[4.05772665830295e-07 -7.83285059789075e-08 -7.83285016498931e-08;-7.83285059789075e-08 4.05772632089447e-07 -7.83285164513028e-08;-7.83285016498931e-08 -7.83285164513028e-08 4.05772808751434e-07]  x1=[0.317544008612314 6568.80905225351 6568.86681609737;314.159265358979 314.159265358979 314.159265358979;0.746603104280062 2.95384642791935 1.38304850173585]  x2=[0.317544219261687 6568.80977399858 6568.86753784894;314.159265358979 314.159265358979 314.159265358979;0.74660175268073 2.95384595122369 1.38304802504009]  x3=[0.00270900047533474 267.644382956312 267.646767069568;314.159265358979 314.159265358979 314.159265358979;0.745450587372901 2.95337741533027 1.38257948909304]  x4=[0.00270900049591147 267.644382971217 267.646767084623;314.159265358979 314.159265358979 314.159265358979;0.74660175763652 2.95384595122302 1.38304802503957]  x5=3.66643048610338e-06  V1=ones(3,3)  V2=ones(3,3)  I1=ones(3,3)  I2=ones(3,3)  nHarmo=1  Measurements=None  Decoupling=off  VsMag0=0  VrMag0=0  VsAngle0=0  VrAngle0=0  IsMag0=0  IrMag0=0  IsAngle0=0  IrAngle0=0
      settings: SourceProductBaseCode=PS
  Scope 6666c334-0968-4852-9779-94ab5a0da3cf : Scope  NumInputPorts=2
  Scope 8072826a-23ba-4558-b3cc-d08b3134df5b : Scope  NumInputPorts=2
  powergui : spspowerguiLib/powergui  Priority=1  SimulationMode=Phasor  SampleTime=50e-6  frequency=50  Iterations=50  frequencyindice=50  Pbase=100e6  ErrMax=1e-4  UnitsV=kV  UnitsW=MW  buscounter=0  FunctionMessages=off  echomessages=off  EnableUseOfTLC=off  CurrentSourceSwitches=off  DisableSnubberDevices=off  DisableRonSwitches=off  DisableVfSwitches=off  DisplayEquations=off  AutomaticDiscreteSolvers=off  SolverType=Tustin/Backward Euler (TBE)  Interpol=off  ExternalGateDelay=off  methode=off  Ts=10  x0status=blocks  SPID=off  SwTol=0  HookPort=off  NonlinearTolerance=1e-4  nMaxIteration=100  ContinueOnMaxIteration=off  RestoreLinks=warning  ResistiveCurrentMeasurement=off  Frange=[0:2:500]  Ylog=off  Xlog=on  ShowGrid=off  save=off  variable=ZData  structure=0  ZoomFFT=off  StartTime=0.0  cycles=1  DisplayStyle=1  fundamental=60  FreqAxis=off  MaxFrequency=1000  frequencyindicesteady=1  RmsSteady=1  display=off
  трансформатор Т-1_ЗТП-1073 : spsThreePhaseSeriesRLCLoadLib/Three-Phase Series RLC Load  Description=Device type: [LOAD], in DispatcherName: [трансформатор Т-1_ЗТП-1073]  LConnTagsString=A|B|C  Configuration=Delta  NominalVoltage=10500  Vabc=[1e3 1e3 1e3]  Vabcp=[1e3 1e3 1e3]  NominalFrequency=50  UnbalancedPower=off  ActivePower=45600  InductivePower=14987.995  CapacitivePower=0  Pabc=[10e3 9e3 11e3]  QLabc=[100 90 110]  QCabc=[100 90 110]  Pabcp=[10e3 9e3 11e3]  QLabcp=[100 90 110]  QCabcp=[100 90 110]  Measurements=None  LoadType=constant Z
  трансформатор Т-1_ЗТП-377 : spsThreePhaseSeriesRLCLoadLib/Three-Phase Series RLC Load  Description=Device type: [LOAD], in DispatcherName: [трансформатор Т-1_ЗТП-377]  LConnTagsString=A|B|C  Configuration=Delta  NominalVoltage=10500  Vabc=[1e3 1e3 1e3]  Vabcp=[1e3 1e3 1e3]  NominalFrequency=50  UnbalancedPower=off  ActivePower=53200  InductivePower=17485.994  CapacitivePower=0  Pabc=[10e3 9e3 11e3]  QLabc=[100 90 110]  QCabc=[100 90 110]  Pabcp=[10e3 9e3 11e3]  QLabcp=[100 90 110]  QCabcp=[100 90 110]  Measurements=None  LoadType=constant Z
  трансформатор Т-2_ЗТП-1073 : spsThreePhaseSeriesRLCLoadLib/Three-Phase Series RLC Load  Description=Device type: [LOAD], in DispatcherName: [трансформатор Т-2_ЗТП-1073]  LConnTagsString=A|B|C  Configuration=Delta  NominalVoltage=10500  Vabc=[1e3 1e3 1e3]  Vabcp=[1e3 1e3 1e3]  NominalFrequency=50  UnbalancedPower=off  ActivePower=45600  InductivePower=14987.995  CapacitivePower=0  Pabc=[10e3 9e3 11e3]  QLabc=[100 90 110]  QCabc=[100 90 110]  Pabcp=[10e3 9e3 11e3]  QLabcp=[100 90 110]  QCabcp=[100 90 110]  Measurements=None  LoadType=constant Z
  трансформатор Т-2_ЗТП-377 : spsThreePhaseSeriesRLCLoadLib/Three-Phase Series RLC Load  Description=Device type: [LOAD], in DispatcherName: [трансформатор Т-2_ЗТП-377]  LConnTagsString=A|B|C  Configuration=Delta  NominalVoltage=10500  Vabc=[1e3 1e3 1e3]  Vabcp=[1e3 1e3 1e3]  NominalFrequency=50  UnbalancedPower=off  ActivePower=53200  InductivePower=17485.994  CapacitivePower=0  Pabc=[10e3 9e3 11e3]  QLabc=[100 90 110]  QCabc=[100 90 110]  Pabcp=[10e3 9e3 11e3]  QLabcp=[100 90 110]  QCabcp=[100 90 110]  Measurements=None  LoadType=constant Z
  трансформатор Т_КТП-1342 : spsThreePhaseSeriesRLCLoadLib/Three-Phase Series RLC Load  Description=Device type: [LOAD], in DispatcherName: [трансформатор Т_КТП-1342]  LConnTagsString=A|B|C  Configuration=Delta  NominalVoltage=10500  Vabc=[1e3 1e3 1e3]  Vabcp=[1e3 1e3 1e3]  NominalFrequency=50  UnbalancedPower=off  ActivePower=1995  InductivePower=655.725  CapacitivePower=0  Pabc=[10e3 9e3 11e3]  QLabc=[100 90 110]  QCabc=[100 90 110]  Pabcp=[10e3 9e3 11e3]  QLabcp=[100 90 110]  QCabcp=[100 90 110]  Measurements=None  LoadType=constant Z
  трансформатор Т_КТП-389 : spsThreePhaseSeriesRLCLoadLib/Three-Phase Series RLC Load  Description=Device type: [LOAD], in DispatcherName: [трансформатор Т_КТП-389]  LConnTagsString=A|B|C  Configuration=Delta  NominalVoltage=10500  Vabc=[1e3 1e3 1e3]  Vabcp=[1e3 1e3 1e3]  NominalFrequency=50  UnbalancedPower=off  ActivePower=90972  InductivePower=29901.05  CapacitivePower=0  Pabc=[10e3 9e3 11e3]  QLabc=[100 90 110]  QCabc=[100 90 110]  Pabcp=[10e3 9e3 11e3]  QLabcp=[100 90 110]  QCabcp=[100 90 110]  Measurements=None  LoadType=constant Z
  wires:
  8072826a-23ba-4558-b3cc-d08b3134df5b/1 -> Scope 8072826a-23ba-4558-b3cc-d08b3134df5b/1
  8072826a-23ba-4558-b3cc-d08b3134df5b/2 -> Scope 8072826a-23ba-4558-b3cc-d08b3134df5b/2
  6666c334-0968-4852-9779-94ab5a0da3cf/1 -> Scope 6666c334-0968-4852-9779-94ab5a0da3cf/1
  6666c334-0968-4852-9779-94ab5a0da3cf/2 -> Scope 6666c334-0968-4852-9779-94ab5a0da3cf/2
  connections:
  трансформатор Т-2_ЗТП-377/LConn1 -- Line 011b7135-821d-4d95-bc11-3e72dddd44ae/RConn1
  трансформатор Т-2_ЗТП-377/LConn2 -- Line 011b7135-821d-4d95-bc11-3e72dddd44ae/RConn2
  трансформатор Т-2_ЗТП-377/LConn3 -- Line 011b7135-821d-4d95-bc11-3e72dddd44ae/RConn3
  Line f1c9c718-c36b-41ce-b023-8d4f642f603e/LConn1 -- Line c3bd0772-1c61-4059-90cf-b754e0a17fa2/RConn1
  Line f1c9c718-c36b-41ce-b023-8d4f642f603e/LConn2 -- Line c3bd0772-1c61-4059-90cf-b754e0a17fa2/RConn2
  Line f1c9c718-c36b-41ce-b023-8d4f642f603e/LConn3 -- Line c3bd0772-1c61-4059-90cf-b754e0a17fa2/RConn3
  6666c334-0968-4852-9779-94ab5a0da3cf/LConn1 -- Line -1257556428/RConn1
  6666c334-0968-4852-9779-94ab5a0da3cf/LConn2 -- Line -1257556428/RConn2
  6666c334-0968-4852-9779-94ab5a0da3cf/LConn3 -- Line -1257556428/RConn3
  трансформатор Т-1_ЗТП-1073/LConn1 -- Line 1e7def22-dd71-47a8-aeb6-b820dd984e65/RConn1
  трансформатор Т-1_ЗТП-1073/LConn2 -- Line 1e7def22-dd71-47a8-aeb6-b820dd984e65/RConn2
  трансформатор Т-1_ЗТП-1073/LConn3 -- Line 1e7def22-dd71-47a8-aeb6-b820dd984e65/RConn3
  трансформатор Т-2_ЗТП-1073/LConn1 -- Line 29ecd01e-d271-4388-90e1-f3eea1c5d3e5/RConn1
  трансформатор Т-2_ЗТП-1073/LConn2 -- Line 29ecd01e-d271-4388-90e1-f3eea1c5d3e5/RConn2
  трансформатор Т-2_ЗТП-1073/LConn3 -- Line 29ecd01e-d271-4388-90e1-f3eea1c5d3e5/RConn3
  Line 687c6ab8-3be1-480c-a391-1a50fba3e886/RConn1 -- Line 1e7def22-dd71-47a8-aeb6-b820dd984e65/LConn1 -- Line 29ecd01e-d271-4388-90e1-f3eea1c5d3e5/LConn1
  Line 687c6ab8-3be1-480c-a391-1a50fba3e886/RConn2 -- Line 1e7def22-dd71-47a8-aeb6-b820dd984e65/LConn2 -- Line 29ecd01e-d271-4388-90e1-f3eea1c5d3e5/LConn2
  Line 687c6ab8-3be1-480c-a391-1a50fba3e886/RConn3 -- Line 1e7def22-dd71-47a8-aeb6-b820dd984e65/LConn3 -- Line 29ecd01e-d271-4388-90e1-f3eea1c5d3e5/LConn3
  Line 566348843/RConn1 -- Line -1257556428/LConn1 -- Line 687c6ab8-3be1-480c-a391-1a50fba3e886/LConn1
  Line 566348843/RConn2 -- Line -1257556428/LConn2 -- Line 687c6ab8-3be1-480c-a391-1a50fba3e886/LConn2
  Line 566348843/RConn3 -- Line -1257556428/LConn3 -- Line 687c6ab8-3be1-480c-a391-1a50fba3e886/LConn3
  трансформатор Т_КТП-389/LConn1 -- Line 5fe16979-df1f-4ffc-8e8c-eea579151a4f/RConn1
  трансформатор Т_КТП-389/LConn2 -- Line 5fe16979-df1f-4ffc-8e8c-eea579151a4f/RConn2
  трансформатор Т_КТП-389/LConn3 -- Line 5fe16979-df1f-4ffc-8e8c-eea579151a4f/RConn3
  Line 1362246896/RConn1 -- Line 566348843/LConn1 -- Line 5fe16979-df1f-4ffc-8e8c-eea579151a4f/LConn1
  Line 1362246896/RConn2 -- Line 566348843/LConn2 -- Line 5fe16979-df1f-4ffc-8e8c-eea579151a4f/LConn2
  Line 1362246896/RConn3 -- Line 566348843/LConn3 -- Line 5fe16979-df1f-4ffc-8e8c-eea579151a4f/LConn3
  Line -379141262/RConn1 -- Line 1362246896/LConn1 -- Line 212fda6c-5c09-4b8e-bb25-d7d47f26dcc3/LConn1
  Line -379141262/RConn2 -- Line 1362246896/LConn2 -- Line 212fda6c-5c09-4b8e-bb25-d7d47f26dcc3/LConn2
  Line -379141262/RConn3 -- Line 1362246896/LConn3 -- Line 212fda6c-5c09-4b8e-bb25-d7d47f26dcc3/LConn3
  трансформатор Т_КТП-1342/LConn1 -- Line d60e7ae4-54f0-4b2e-a601-9678671982ab/RConn1
  трансформатор Т_КТП-1342/LConn2 -- Line d60e7ae4-54f0-4b2e-a601-9678671982ab/RConn2
  трансформатор Т_КТП-1342/LConn3 -- Line d60e7ae4-54f0-4b2e-a601-9678671982ab/RConn3
  Line 2120786381/RConn1 -- Line -379141262/LConn1 -- Line d60e7ae4-54f0-4b2e-a601-9678671982ab/LConn1
  Line 2120786381/RConn2 -- Line -379141262/LConn2 -- Line d60e7ae4-54f0-4b2e-a601-9678671982ab/LConn2
  Line 2120786381/RConn3 -- Line -379141262/LConn3 -- Line d60e7ae4-54f0-4b2e-a601-9678671982ab/LConn3
  Line e9a22d10-c169-4cb9-b823-11c73169328c/RConn1 -- Line -346508084/LConn1 -- Line 2120786381/LConn1
  Line e9a22d10-c169-4cb9-b823-11c73169328c/RConn2 -- Line -346508084/LConn2 -- Line 2120786381/LConn2
  Line e9a22d10-c169-4cb9-b823-11c73169328c/RConn3 -- Line -346508084/LConn3 -- Line 2120786381/LConn3
  Line 1716516389/RConn1 -- Line 89d3125f-fc75-4299-8889-5174924ee4ad/LConn1 -- Line c3bd0772-1c61-4059-90cf-b754e0a17fa2/LConn1 -- Line e9a22d10-c169-4cb9-b823-11c73169328c/LConn1
  Line 1716516389/RConn2 -- Line 89d3125f-fc75-4299-8889-5174924ee4ad/LConn2 -- Line c3bd0772-1c61-4059-90cf-b754e0a17fa2/LConn2 -- Line e9a22d10-c169-4cb9-b823-11c73169328c/LConn2
  Line 1716516389/RConn3 -- Line 89d3125f-fc75-4299-8889-5174924ee4ad/LConn3 -- Line c3bd0772-1c61-4059-90cf-b754e0a17fa2/LConn3 -- Line e9a22d10-c169-4cb9-b823-11c73169328c/LConn3
  трансформатор Т-1_ЗТП-377/LConn1 -- Line 2b3928e6-1e74-4724-a381-14e26628662e/RConn1
  трансформатор Т-1_ЗТП-377/LConn2 -- Line 2b3928e6-1e74-4724-a381-14e26628662e/RConn2
  трансформатор Т-1_ЗТП-377/LConn3 -- Line 2b3928e6-1e74-4724-a381-14e26628662e/RConn3
  Line 285053675/RConn1 -- Line 011b7135-821d-4d95-bc11-3e72dddd44ae/LConn1 -- Line 1716516389/LConn1 -- Line 2b3928e6-1e74-4724-a381-14e26628662e/LConn1
  Line 285053675/RConn2 -- Line 011b7135-821d-4d95-bc11-3e72dddd44ae/LConn2 -- Line 1716516389/LConn2 -- Line 2b3928e6-1e74-4724-a381-14e26628662e/LConn2
  Line 285053675/RConn3 -- Line 011b7135-821d-4d95-bc11-3e72dddd44ae/LConn3 -- Line 1716516389/LConn3 -- Line 2b3928e6-1e74-4724-a381-14e26628662e/LConn3
  Line 458366992/RConn1 -- Line 285053675/LConn1 -- Line 867f1459-8b81-4976-9bab-74549e53d0e3/LConn1
  Line 458366992/RConn2 -- Line 285053675/LConn2 -- Line 867f1459-8b81-4976-9bab-74549e53d0e3/LConn2
  Line 458366992/RConn3 -- Line 285053675/LConn3 -- Line 867f1459-8b81-4976-9bab-74549e53d0e3/LConn3
  Line 458366992/LConn1 -- 8072826a-23ba-4558-b3cc-d08b3134df5b/RConn1
  Line 458366992/LConn2 -- 8072826a-23ba-4558-b3cc-d08b3134df5b/RConn2
  Line 458366992/LConn3 -- 8072826a-23ba-4558-b3cc-d08b3134df5b/RConn3
